simulink model "vector_gain_ref"  (R2020b)
settings: Solver=FixedStepDiscrete  StartTime=0.0  StopTime=stopTime  RelTol=1e-3
settings Model: Creator=Ross  LastModifiedBy=wickh
settings SolverCC: AutoInsertRateTranBlk=on
settings DataIOCC: SaveOutput=off  SaveTime=off  ReturnWorkspaceOutputs=off
settings OptimizationCC: BlockReduction=off  ConditionallyExecuteInputs=off  DefaultParameterBehavior=Inlined
settings DebuggingCC: SignalInfNanChecking=error  SignalRangeChecking=warning  ReadBeforeWriteMsg=DisableAll  WriteAfterWriteMsg=DisableAll  WriteAfterReadMsg=DisableAll  AlgebraicLoopMsg=error  MultiTaskDSMMsg=none  SingleTaskRateTransMsg=error  ParameterUnderflowMsg=warning  UnderSpecifiedDataTypeMsg=error  PregeneratedLibrarySubsystemCodeDiagnostic=none  ArithmeticOperatorsInVariantConditions=warning
settings HardwareCC: ProdBitPerPointer=32  ProdBitPerSizeT=32  ProdBitPerPtrDiffT=32  ProdLargestAtomicFloat=None  ProdIntDivRoundTo=Undefined  ProdEndianess=Unspecified  ProdWordSize=32  ProdHWDeviceType=ASIC/FPGA->ASIC/FPGA  TargetBitPerPointer=64  TargetBitPerSizeT=64  TargetBitPerPtrDiffT=64  TargetLongLongMode=on  TargetIntDivRoundTo=Zero  TargetEndianess=LittleEndian  TargetWordSize=64  TargetHWDeviceType=Custom Processor->MATLAB Host Computer  ProdEqTarget=off
settings ModelReferenceCC: UpdateModelReferenceTargets=IfOutOfDate
settings SFSimCC: SFSimEcho=off  SimUseLocalCustomCode=off  CustomCodeUndefinedFunction=UseInterfaceOnly
settings RTWCC: RTWUseLocalCustomCode=off

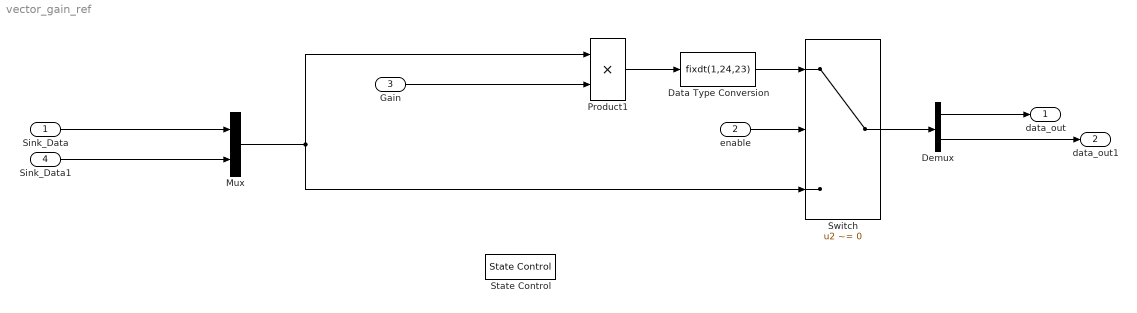
== system vector_gain_ref ==
  Sink_Data : Inport  OutDataTypeStr=fixdt(1,24,23)  PortDimensions=1
  enable : Inport  Port=2  OutDataTypeStr=boolean  PortDimensions=1
  Gain : Inport  Port=3  OutDataTypeStr=gain_dt  PortDimensions=1
  Sink_Data1 : Inport  Port=4  OutDataTypeStr=fixdt(1,24,23)  PortDimensions=1
  Data Type Conversion : DataTypeConversion  OutDataTypeStr=fixdt(1,24,23)
  Demux : Demux  Outputs=2
  Mux : Mux  Inputs=2
  Product1 : Product
  State Control : StateControl  StateControl=Synchronous
  Switch : Switch  Criteria=u2 ~= 0
  data_out : Outport  OutDataTypeStr=fixdt(1,24,23)  PortDimensions=1
  data_out1 : Outport  Port=2  OutDataTypeStr=fixdt(1,24,23)  PortDimensions=1
  wires:
  Data Type Conversion/1 -> Switch/1
  Product1/1 -> Data Type Conversion/1
  Gain/1 -> Product1/2
  Sink_Data/1 -> Mux/1
  enable/1 -> Switch/2
  Sink_Data1/1 -> Mux/2
  Mux/1 -> Switch/3, Product1/1
  Switch/1 -> Demux/1
  Demux/2 -> data_out1/1
  Demux/1 -> data_out/1
